simulink model "test07"  (R2021a)
settings: Solver=VariableStepAuto  StartTime=0.0  StopTime=20  RelTol=1e-3
libraries: HORTISIM x8
settings Model: Creator=djoroya  LastModifiedBy=djoroya
settings DebuggingCC: UnconnectedInputMsg=none  UnconnectedOutputMsg=none  UnconnectedLineMsg=none

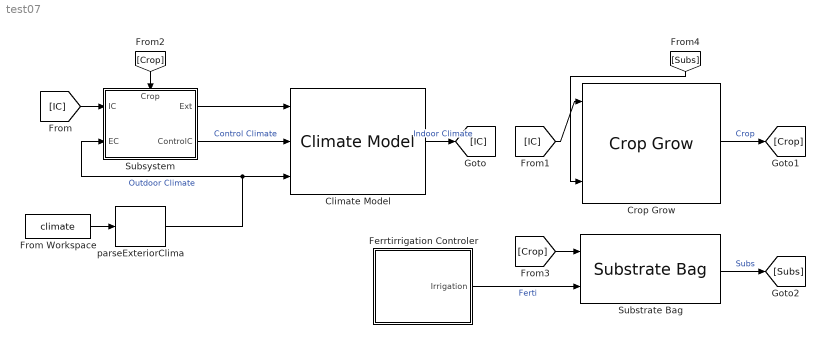
== system test07 ==
  Climate Model : HORTISIM/Climate/Models/Climate Model  params=params  x0=cic
      settings: SourceProductName=Horti Simulator
  Crop Grow : HORTISIM/Horticulture/Models/Crop Grow  params=crop_params  x0=x0_crop
      settings: SourceProductName=Horti Simulator
  Ferrtirrigation Controler : Subsystem  AncestorBlock="HORTISIM/Horticulture/Controls/Ferrtirrigation  Controler"
      mask Display: image('$imagefile'); % Use "Edit Image" on toolstrip to change.
  From Workspace : FromWorkspace  VariableName=climate
  Substrate Bag : HORTISIM/Horticulture/Models/Substrate Bag  x0=x0_substrate  params=substrate_params
      settings: SourceProductName=Horti Simulator
  Subsystem : Subsystem
      settings: PortSchema="{\"entries\":[{\"content\":{\"sides\":[{\"content\":{\"connectorIds\":[\"In1\",\"In2\"]},\"type\":\"ConnectorPlacement.EquallySpacedRectSide\",\"uuid\":\"05a20284-31f0-4954-ac42-b08c051c723b\"},{\"content\":{\"connectorIds\":[\"Out1\",\"Out2\"],\"side\":\"RIGHT\"},\"type\":\"ConnectorPlacement.EquallySpacedRectSide\",\"uuid\":\"7e4ab434-6629-473e-82a5-f81f17f0ab6e\"},{\"content\":{\"connectorIds\":[\"In3\"],\"side\":\"TOP\"},\"type\":\"ConnectorPlacement.EquallySpacedRectSide\",\"uuid\":\"2ea64524-8947-456a-a977-2c05776eabaa\"}]},\"type\":\"ConnectorPlacement.EquallySpacedConnector\",\"uuid\":\"6035ded9-300f-4f3c-adde-f9d2e7ea6cf9\"}],\"packageUris\":[\"http://schema.mathworks.com/mf0/Connector/R2020b\"],\"version\":\"1.0\"}"
  parseExteriorClima : HORTISIM/Other  Functions/parseExteriorClima  SystemSampleTime=-1  VariantActivationTime=update diagram  Latency=0  AutoFrameSizeCalculation=off
      settings: SourceProductName=Horti Simulator
  wires:
  From Workspace/1 -> parseExteriorClima/1
  parseExteriorClima/1 -> Climate Model/3, Subsystem/2(EC)  "Outdoor Climate"
  Climate Model/1 -> [IC]  "Indoor Climate"
  Subsystem/2(ControlC) -> Climate Model/2  "Control Climate"
  [IC] -> Subsystem/1(IC)
  Subsystem/1(Ext) -> Climate Model/1
  [IC] -> Crop Grow/1
  Crop Grow/1 -> [Crop]  "Crop"
  [Crop] -> Subsystem/3(Crop)
  [Crop] -> Substrate Bag/1
  Substrate Bag/1 -> [Subs]  "Subs"
  [Subs] -> Crop Grow/3
  Ferrtirrigation Controler/1(Irrigation) -> Substrate Bag/2  "Ferti"

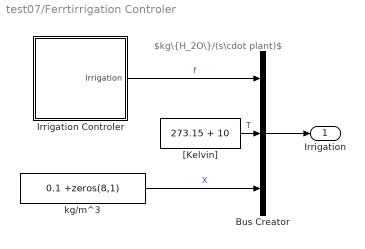
== system test07/Ferrtirrigation Controler ==
  note: $kg\{H_2O\}/(s\cdot plant)$
  Bus Creator : BusCreator  Inputs=3  OutDataTypeStr=Bus: FLOW  NonVirtualBus=on
  Irrigation Controler : Subsystem
  "[Kelvin]" : Constant  Value=273.15 + 10
  kg/m^3 : Constant  Value=0.1 +zeros(8,1)
  Irrigation : Outport
  wires:
  kg/m^3/1 -> Bus Creator/3  "X"
  Irrigation Controler/1(Irrigation) -> Bus Creator/1  "f"
  "[Kelvin]"/1 -> Bus Creator/2  "T"
  Bus Creator/1 -> Irrigation/1

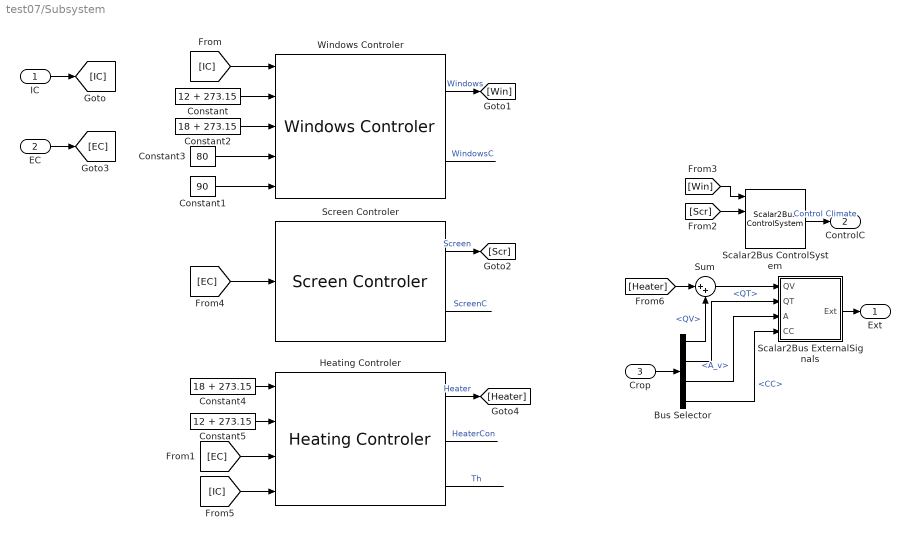
== system test07/Subsystem ==
  IC : Inport
  EC : Inport  Port=2
  Crop : Inport  Port=3
  Bus Selector : BusSelector  OutputSignals=HeatVars.QV,HeatVars.QT,A_v,CC
  Constant : Constant  Value=12 + 273.15
  Constant1 : Constant  Value=90
  Constant2 : Constant  Value=18 + 273.15
  Constant3 : Constant  Value=80
  Constant4 : Constant  Value=18 + 273.15
  Constant5 : Constant  Value=12 + 273.15
  Heating Controler : HORTISIM/Climate/Controls/Heating Controler  params=heat_p  x0=heat_ic
      settings: SourceProductName=Horti Simulator
  Scalar2Bus ControlSystem : HORTISIM/Other  Functions/Scalar2Bus  ControlSystem  SystemSampleTime=-1  VariantActivationTime=update diagram  Latency=0  AutoFrameSizeCalculation=off
      settings: SourceProductName=Horti Simulator
  Scalar2Bus ExternalSignals : Subsystem
  Screen Controler : HORTISIM/Climate/Controls/Screen Controler  params=scr_p
      settings: SourceProductName=Horti Simulator
  Sum : Sum  Inputs=|++
  Windows Controler : HORTISIM/Climate/Controls/Windows Controler  params=win_p
      settings: SourceProductName=Horti Simulator
  Ext : Outport
  ControlC : Outport  Port=2
  wires:
  Constant2/1 -> Windows Controler/3
  Constant3/1 -> Windows Controler/4
  Windows Controler/2 -> ?  "WindowsC"
  Constant1/1 -> Windows Controler/5
  Constant/1 -> Windows Controler/2
  IC/1 -> [IC]
  [IC] -> Windows Controler/1
  Windows Controler/1 -> [Win]  "Windows"
  Screen Controler/1 -> [Scr]  "Screen"
  [Scr] -> Scalar2Bus ControlSystem/2
  [Win] -> Scalar2Bus ControlSystem/1
  Scalar2Bus ControlSystem/1 -> ControlC/1  "Control Climate"
  EC/1 -> [EC]
  [EC] -> Screen Controler/1
  Screen Controler/2 -> ?  "ScreenC"
  [EC] -> Heating Controler/3
  [IC] -> Heating Controler/4
  Constant4/1 -> Heating Controler/1
  Constant5/1 -> Heating Controler/2
  Heating Controler/1 -> [Heater]  "Heater"
  Scalar2Bus ExternalSignals/1(Ext) -> Ext/1
  Heating Controler/3 -> ?  "Th"
  Heating Controler/2 -> ?  "HeaterCon"
  Crop/1 -> Bus Selector/1
  Bus Selector/2 -> Scalar2Bus ExternalSignals/2(QT)  "<QT>"
  [Heater] -> Sum/1
  Sum/1 -> Scalar2Bus ExternalSignals/1(QV)
  Bus Selector/1 -> Sum/2  "<QV>"
  Bus Selector/3 -> Scalar2Bus ExternalSignals/3(A)  "<A_v>"
  Bus Selector/4 -> Scalar2Bus ExternalSignals/4(CC)  "<CC>"

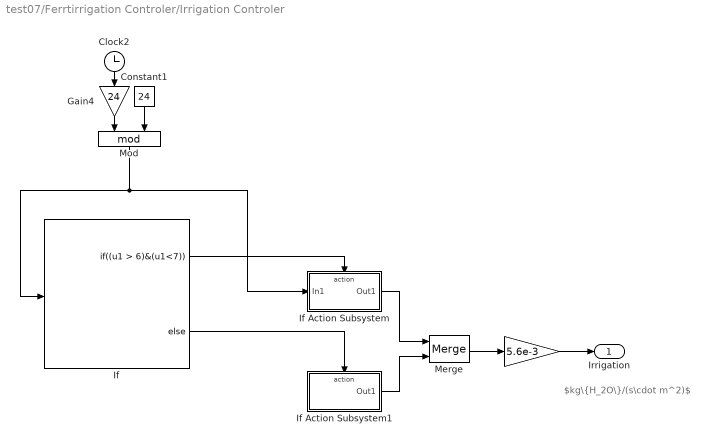
== system test07/Ferrtirrigation Controler/Irrigation Controler ==
  note: $kg\{H_2O\}/(s\cdot m^2)$
  " " : Gain  Gain=5.6e-3
  Clock2 : Clock
  Constant1 : Constant  Value=24
  Gain4 : Gain  Gain=24
  If : If  IfExpression=(u1 > 6)&(u1<7)
  If Action Subsystem : Subsystem  TreatAsAtomicUnit=on
  If Action Subsystem1 : Subsystem  TreatAsAtomicUnit=on
  Merge : Merge
  Mod : Math  Operator=mod  SaturateOnIntegerOverflow=on
  Irrigation : Outport
  wires:
  Merge/1 -> " "/1
  If Action Subsystem1/1(Out1) -> Merge/2
  If Action Subsystem/1(Out1) -> Merge/1
  If/2 -> If Action Subsystem1/Action
  If/1 -> If Action Subsystem/Action
  Mod/1 -> If Action Subsystem/1(In1), If/1
  Gain4/1 -> Mod/1
  Clock2/1 -> Gain4/1
  Constant1/1 -> Mod/2
  " "/1 -> Irrigation/1

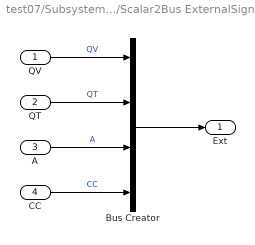
== system test07/Subsystem/Scalar2Bus ExternalSignals ==
  QV : Inport
  QT : Inport  Port=2
  A : Inport  Port=3
  CC : Inport  Port=4
  Bus Creator : BusCreator  Inputs=4
  Ext : Outport
  wires:
  QT/1 -> Bus Creator/2  "QT"
  QV/1 -> Bus Creator/1  "QV"
  A/1 -> Bus Creator/3  "A"
  CC/1 -> Bus Creator/4  "CC"
  Bus Creator/1 -> Ext/1

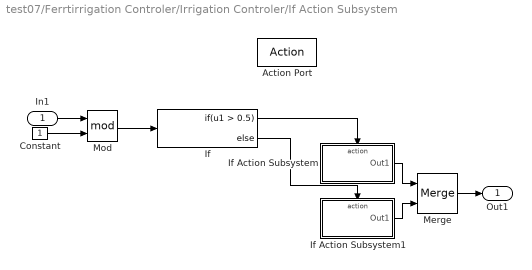
== system test07/Ferrtirrigation Controler/Irrigation Controler/If Action Subsystem ==
  In1 : Inport
  Action Port : ActionPort  ActionPortLabel=if((u1 > 6)&(u1<7))
  Constant : Constant
  If : If  IfExpression=u1 > 0.5
  If Action Subsystem : Subsystem  TreatAsAtomicUnit=on
  If Action Subsystem1 : Subsystem  TreatAsAtomicUnit=on
  Merge : Merge
  Mod : Math  Operator=mod  SaturateOnIntegerOverflow=on
  Out1 : Outport
  wires:
  Merge/1 -> Out1/1
  If Action Subsystem1/1(Out1) -> Merge/2
  If Action Subsystem/1(Out1) -> Merge/1
  If/2 -> If Action Subsystem1/Action
  If/1 -> If Action Subsystem/Action
  Mod/1 -> If/1
  Constant/1 -> Mod/2
  In1/1 -> Mod/1

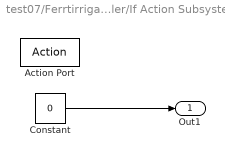
== system test07/Ferrtirrigation Controler/Irrigation Controler/If Action Subsystem1 ==
  Action Port : ActionPort  ActionPortLabel=else
  Constant : Constant  Value=0
  Out1 : Outport
  wires:
  Constant/1 -> Out1/1

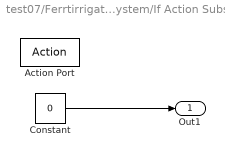
== system test07/Ferrtirrigation Controler/Irrigation Controler/If Action Subsystem/If Action Subsystem ==
  Action Port : ActionPort  ActionPortLabel=if(u1 > 0.5)
  Constant : Constant  Value=0
  Out1 : Outport
  wires:
  Constant/1 -> Out1/1

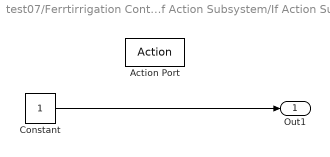
== system test07/Ferrtirrigation Controler/Irrigation Controler/If Action Subsystem/If Action Subsystem1 ==
  Action Port : ActionPort  ActionPortLabel=else
  Constant : Constant
  Out1 : Outport
  wires:
  Constant/1 -> Out1/1
